simulink model "PID_Homework_Hong"  (R2024b)
settings: Solver=VariableStepAuto  StartTime=0.0  StopTime=100  RelTol=1e-3
(part 2 of 2)

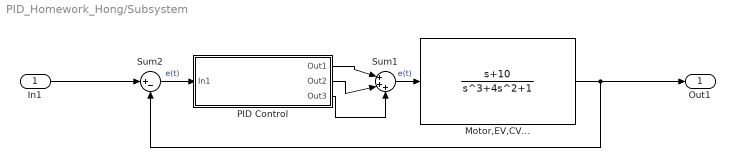
== system PID_Homework_Hong/Subsystem ==
  In1 : Inport
  Motor,EV,CV... : TransferFcn  Numerator=[1 10]  Denominator=[1 4 0 1]
  PID Control : Subsystem
  Sum1 : Sum  Inputs=|+++
  Sum2 : Sum  Inputs=|+-
  Out1 : Outport
  wires:
  Motor,EV,CV.../1 -> Out1/1, Sum2/2
  PID Control/3(Out3) -> Sum1/3
  Sum1/1 -> Motor,EV,CV.../1  "e(t)"
  Sum2/1 -> PID Control/1(In1)  "e(t)"
  PID Control/1(Out1) -> Sum1/1
  In1/1 -> Sum2/1
  PID Control/2(Out2) -> Sum1/2

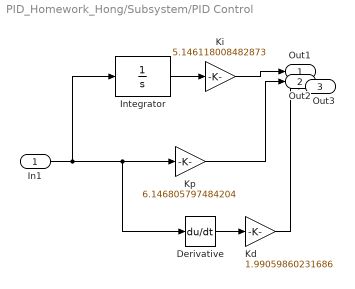
== system PID_Homework_Hong/Subsystem/PID Control ==
  In1 : Inport
  Derivative : Derivative
  Integrator : Integrator
  Kd : Gain  Gain=1.99059860231686
  Ki : Gain  Gain=5.146118008482873
  Kp : Gain  Gain=6.146805797484204
  Out1 : Outport
  Out2 : Outport  Port=2
  Out3 : Outport  Port=3
  wires:
  Integrator/1 -> Ki/1
  In1/1 -> Integrator/1, Derivative/1, Kp/1
  Derivative/1 -> Kd/1
  Kd/1 -> Out3/1
  Ki/1 -> Out1/1
  Kp/1 -> Out2/1
